simulink model "Simulator"  (R2024b)
settings: Solver=FixedStepAuto  StartTime=0.0  StopTime=Parameters.Simulink.sim_time_s  FixedStep=Parameters.Simulink.time_step_s  RelTol=1e-6
undefined symbols (not defined in the file): att_0, data, flight_mode, FLIGHT_MODE, id, joystick, Parameters, res, timestamp, traj_opt, wait_time_s
libraries: dspsigops x3, simulink x2, eeGeneralControl x2, px4uORBlib x2, vrlib x1, simulink_extras x1, aerolibanimutils x1, sharedtransform x1
(part 1 of 2)
settings Model: DataDictionary=simulink_data_types.sldd  Creator=thesa  LastModifiedBy=thesa
settings SolverCC: EnableFixedStepZeroCrossing=on
settings RTWCC: GPUComputeCapability=3.5

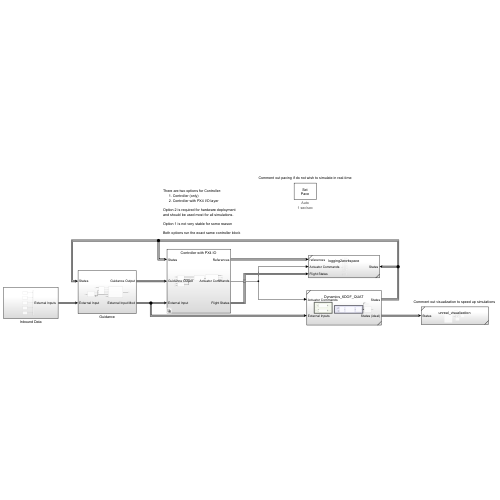
[thumbnail: Simulink's stored preview of the top-level diagram]
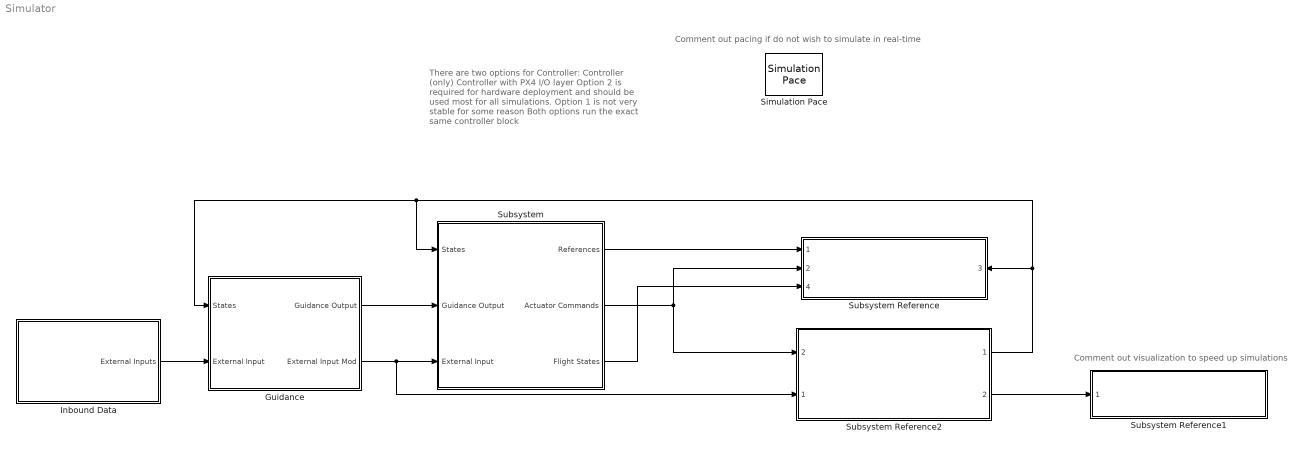
== system Simulator ==
  note: There are two options for Controller:
      | Controller (only)
      | Controller with PX4 I/O layer
      |
      | Option 2 is required for hardware deployment
      | and should be used most for all simulations.
      |
      | Option 1 is not very stable for some reason
      |
      | Both options run the exact same controller block
  note: Comment out pacing if do not wish to simulate in real-time
  note: Comment out visualization to speed up simulations
  Guidance : Subsystem
  Inbound Data : Subsystem
  Simulation Pace : aerolibanimutils/Simulation Pace  SimulationPace=1  SleepMode=Auto  OutputPaceError=off  SampleTime=-1
  Subsystem : Subsystem  Variant=on  VariantControlMode=label  VariantControl=Choice  LabelModeActiveChoice=Choice_1
  Subsystem Reference : Subsystem  ReferencedSubsystem=logging2workspace
      settings: PortSchema="{\"entries\":[{\"content\":{\"sides\":[{\"content\":{\"connectorIds\":[\"In1\",\"In2\",\"In4\"]},\"type\":\"ConnectorPlacement.EquallySpacedRectSide\",\"uuid\":\"47b0435c-4974-4dfb-aae6-6ca620e26367\"},{\"content\":{\"connectorIds\":[\"In3\"],\"side\":\"RIGHT\"},\"type\":\"ConnectorPlacement.EquallySpacedRectSide\",\"uuid\":\"e323305f-4ea2-4fd9-9ec2-838e165181fb\"},{\"content\":{\"side\":\"TOP\"},\"type\":\"ConnectorPlacement.EquallySpacedRectSide\",\"uuid\":\"bec00405-cbc9-4439-89df-ad1a7655b850\"}]},\"type\":\"ConnectorPlacement.EquallySpacedConnector\",\"uuid\":\"1e7e1f21-3d1e-40b5-a907-670aed2a63f6\"}],\"packageUris\":[\"http://schema.mathworks.com/mf0/Connector/R2020b\"],\"version\":\"1.0\"}"
  Subsystem Reference1 : Subsystem  ReferencedSubsystem=unreal_visualization
  Subsystem Reference2 : Subsystem  ReferencedSubsystem=Dynamics_6DOF_QUAT
      settings: PortSchema="{\"entries\":[{\"content\":{\"sides\":[{\"content\":{\"connectorIds\":[\"In2\",\"In1\"]},\"type\":\"ConnectorPlacement.EquallySpacedRectSide\",\"uuid\":\"67a10377-dfc9-4fe8-a62d-93af2914f52a\"},{\"content\":{\"connectorIds\":[\"Out1\",\"Out2\"],\"side\":\"RIGHT\"},\"type\":\"ConnectorPlacement.EquallySpacedRectSide\",\"uuid\":\"9c2068d6-d6c5-47ba-96fe-f41bc3930446\"},{\"content\":{\"side\":\"TOP\"},\"type\":\"ConnectorPlacement.EquallySpacedRectSide\",\"uuid\":\"c021d50f-d597-4e02-a45a-8416f053316a\"}]},\"type\":\"ConnectorPlacement.EquallySpacedConnector\",\"uuid\":\"5c77a6da-dceb-4faf-ad40-bce586c717c3\"}],\"packageUris\":[\"http://schema.mathworks.com/mf0/Connector/R2020b\"],\"version\":\"1.0\"}"
  wires:
  Inbound Data/1("External Inputs ") -> Guidance/2(External Input)
  Subsystem Reference2/1 -> Subsystem/1(States), Guidance/1(States), Subsystem Reference/3
  Subsystem/1(References) -> Subsystem Reference/1
  Subsystem/2(Actuator Commands) -> Subsystem Reference2/2, Subsystem Reference/2
  Subsystem/3(Flight States) -> Subsystem Reference/4
  Guidance/2(External Input Mod) -> Subsystem Reference2/1, Subsystem/3(External Input)
  Guidance/1(Guidance Output) -> Subsystem/2(Guidance Output)
  Subsystem Reference2/2 -> Subsystem Reference1/1

== system Simulator/Guidance ==
  States : Inport
  External Input : Inport  Port=2
  Guidance Initialization : Subsystem
  States1 : InportShadow
  Subsystem1 : Subsystem
  Subsystem2 : Subsystem  Variant=on  VariantControlMode=label  VariantControl=Choice  LabelModeActiveChoice=Choice
  Guidance Output : Outport
  External Input Mod : Outport  Port=2
  wires:
  Guidance Initialization/4(yaw_0) -> Subsystem2/4(yaw_0)
  Guidance Initialization/2(t) -> Subsystem2/2(time_since_start_of_traj)
  Subsystem2/1(trajectory) -> Guidance Output/1  "trajectory"
  Guidance Initialization/3("p_e_0 ") -> Subsystem2/3(p_e_0)
  States/1 -> Guidance Initialization/1(States)
  External Input/1 -> Subsystem1/1(External Input)
  Subsystem1/2(External Input Mod) -> Subsystem2/5(External Inputs), Guidance Initialization/2(External Input), External Input Mod/1
  Subsystem1/1(reset) -> Guidance Initialization/3(reset)
  States1/1 -> Subsystem2/6(States)
  Guidance Initialization/1(guidance_active) -> Subsystem2/1(guidance_active)

== system Simulator/Inbound Data ==
  Bus Creator3 : BusCreator  Inputs=5
  Subsystem1 : Subsystem
  Subsystem2 : Subsystem
  Subsystem3 : Subsystem
  Subsystem4 : Subsystem
  Subsystem5 : Subsystem
  "External Inputs " : Outport
  wires:
  Bus Creator3/1 -> "External Inputs "/1
  Subsystem1/1(Control Gains) -> Bus Creator3/2  "Control Gains"
  Subsystem2/1(Vehicle Parameters) -> Bus Creator3/1  "Vehicle Parameters"
  Subsystem3/1(Trajectory) -> Bus Creator3/4  "Trajectory"
  Subsystem4/1(Pilot Input) -> Bus Creator3/5  "Pilot Input"
  Subsystem5/1(Control Logic) -> Bus Creator3/3  "Control Logic"

== system Simulator/Subsystem ==
  States : Inport
  Guidance Output : Inport  Port=2
  External Input : Inport  Port=3
  Controller (only) : Subsystem  VariantControl=Controller (only)
  Controller with PX4 IO : Subsystem  VariantControl=Choice_1
  References : Outport
  Actuator Commands : Outport  Port=2
  Flight States : Outport  Port=3

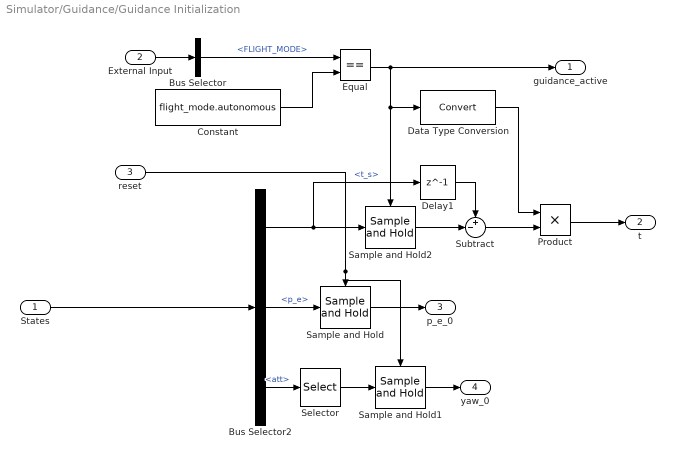
== system Simulator/Guidance/Guidance Initialization ==
  States : Inport
  External Input : Inport  Port=2
  reset : Inport  Port=3
  Bus Selector : BusSelector  OutputSignals=Pilot Input.FLIGHT_MODE
  Bus Selector2 : BusSelector  OutputSignals=t_s,p_e,att
  Constant : Constant  Value=flight_mode.autonomous
  Data Type Conversion : DataTypeConversion  SaturateOnIntegerOverflow=off  RndMeth=Floor
  Delay1 : Delay  DelayLength=1
  Equal : RelationalOperator  Operator===  OutDataTypeStr=boolean  RndMeth=Simplest  InputSameDT=off
  Product : Product
  Sample and Hold : dspsigops/Sample and Hold  trig=Rising edge  initCond=p_0  latchinput=off
  Sample and Hold1 : dspsigops/Sample and Hold  trig=Rising edge  initCond=att_0(3)  latchinput=off
  Sample and Hold2 : dspsigops/Sample and Hold  trig=Rising edge  initCond=0  latchinput=off
  Selector : Selector  InputPortWidth=3  IndexOptions=Index vector (dialog)  Indices=[3]  OutputSizes=1
  Subtract : Sum  Inputs=+-|
  guidance_active : Outport
  t : Outport  Port=2
  "p_e_0 " : Outport  Port=3
  yaw_0 : Outport  Port=4
  wires:
  Delay1/1 -> Subtract/1
  Subtract/1 -> Product/2
  Sample and Hold2/1 -> Subtract/2
  Bus Selector2/1 -> Delay1/1, Sample and Hold2/1  "<t_s>"
  Bus Selector2/3 -> Selector/1  "<att>"
  reset/1 -> Sample and Hold/Trigger, Sample and Hold1/Trigger
  States/1 -> Bus Selector2/1
  Bus Selector2/2 -> Sample and Hold/1  "<p_e>"
  Sample and Hold/1 -> "p_e_0 "/1
  Selector/1 -> Sample and Hold1/1
  Sample and Hold1/1 -> yaw_0/1
  External Input/1 -> Bus Selector/1
  Bus Selector/1 -> Equal/1  "<FLIGHT_MODE>"
  Constant/1 -> Equal/2
  Equal/1 -> guidance_active/1, Data Type Conversion/1, Sample and Hold2/Trigger
  Product/1 -> t/1
  Data Type Conversion/1 -> Product/1

== system Simulator/Guidance/Subsystem1 ==
  External Input : Inport
  Bus Assignment : BusAssignment  AssignedSignals=Pilot Input.FLIGHT_MODE
  Bus Selector : BusSelector  OutputSignals=Pilot Input.Parameters.time_step_s,Pilot Input.Parameters.AUTO_DELAY_S
  Bus Selector4 : BusSelector  OutputSignals=Pilot Input.FLIGHT_MODE
  Delay : Delay  DelayLength=1  InitialCondition=flight_mode.position_hold
  Delay1 : Delay  DelayLength=1
  Delay2 : Delay  DelayLength=1  InitialCondition=false
  Divide : Product  Inputs=*/
  MATLAB Function : MATLAB Function  TreatAsAtomicUnit=on
  reset : Outport
  External Input Mod : Outport  Port=2
  wires:
  MATLAB Function/1(current_mode) -> Delay/1
  External Input/1 -> Bus Assignment/1, Bus Selector4/1, Bus Selector/1
  Divide/1 -> MATLAB Function/4(wait_time)
  Bus Assignment/1 -> External Input Mod/1
  Bus Selector/2 -> Divide/1  "<AUTO_DELAY_S>"
  Bus Selector/1 -> Divide/2  "<time_step_s>"
  MATLAB Function/2(reset) -> Delay2/1
  MATLAB Function/3(timer) -> Delay1/1
  Delay/1 -> Bus Assignment/2, MATLAB Function/2("current_mode ")
  Bus Selector4/1 -> MATLAB Function/1(mode_request)  "<FLIGHT_MODE>"
  Delay1/1 -> MATLAB Function/3("timer ")
  Delay2/1 -> reset/1

== system Simulator/Guidance/Subsystem2 ==
  guidance_active : Inport
  time_since_start_of_traj : Inport  Port=2
  p_e_0 : Inport  Port=3
  yaw_0 : Inport  Port=4
  External Inputs : Inport  Port=5
  States : Inport  Port=6
  Step input : Subsystem  VariantControl=Choice_1
  minimum_snap : Subsystem  VariantControl=Choice
  trajectory : Outport

== system Simulator/Inbound Data/Subsystem1 ==
  " K-matrix control (LQR, H-inf, etc.)" : Subsystem
  Bus Creator2 : BusCreator  Inputs=9
  Constant1 : Constant  Value=Parameters.Control.Gains.K_omega_dot
  Constant13 : Constant  Value=Parameters.Control.Gains.K_omega
  Constant18 : Constant  Value=Parameters.Control.Gains.K_pos_int
  Constant2 : Constant  Value=Parameters.Control.Gains.K_omega_I
  Constant6 : Constant  Value=Parameters.Control.Gains.K_pos
  Constant7 : Constant  Value=Parameters.Control.Gains.K_vel
  Constant8 : Constant  Value=Parameters.Control.Gains.K_att
  Constant9 : Constant  Value=Parameters.Control.Gains.K_acc
  Control Gains : Outport
  wires:
  Constant7/1 -> Bus Creator2/3  "K_vel"
  Constant6/1 -> Bus Creator2/1  "K_pos"
  Constant13/1 -> Bus Creator2/6  "K_omega"
  Bus Creator2/1 -> Control Gains/1  "Control Gains"
  Constant18/1 -> Bus Creator2/2  "K_pos_int"
  Constant9/1 -> Bus Creator2/4  "K_acc"
  Constant8/1 -> Bus Creator2/5  "K_att"
  " K-matrix control (LQR, H-inf, etc.)"/1(K_matrix_control) -> Bus Creator2/9  "K_matrix_control"
  Constant1/1 -> Bus Creator2/8  "K_omega_dot"
  Constant2/1 -> Bus Creator2/7  "K_omega_I"

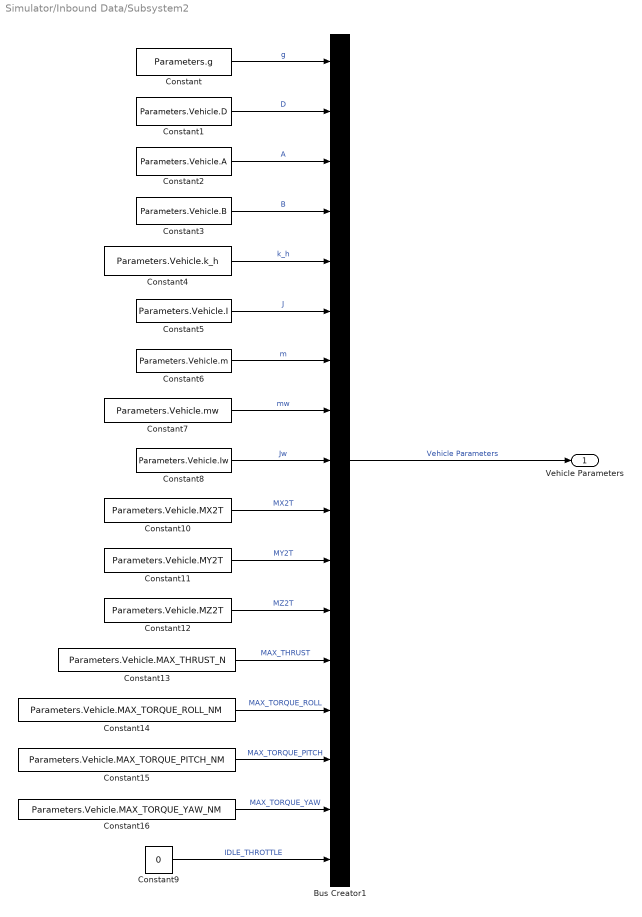
== system Simulator/Inbound Data/Subsystem2 ==
  Bus Creator1 : BusCreator  Inputs=17
  Constant : Constant  Value=Parameters.g
  Constant1 : Constant  Value=Parameters.Vehicle.D
  Constant10 : Constant  Value=Parameters.Vehicle.MX2T
  Constant11 : Constant  Value=Parameters.Vehicle.MY2T
  Constant12 : Constant  Value=Parameters.Vehicle.MZ2T
  Constant13 : Constant  Value=Parameters.Vehicle.MAX_THRUST_N
  Constant14 : Constant  Value=Parameters.Vehicle.MAX_TORQUE_ROLL_NM
  Constant15 : Constant  Value=Parameters.Vehicle.MAX_TORQUE_PITCH_NM
  Constant16 : Constant  Value=Parameters.Vehicle.MAX_TORQUE_YAW_NM
  Constant2 : Constant  Value=Parameters.Vehicle.A
  Constant3 : Constant  Value=Parameters.Vehicle.B
  Constant4 : Constant  Value=Parameters.Vehicle.k_h
  Constant5 : Constant  Value=Parameters.Vehicle.I
  Constant6 : Constant  Value=Parameters.Vehicle.m
  Constant7 : Constant  Value=Parameters.Vehicle.mw
  Constant8 : Constant  Value=Parameters.Vehicle.Iw
  Constant9 : Constant  Value=0
  Vehicle Parameters : Outport
  wires:
  Constant5/1 -> Bus Creator1/6  "J"
  Constant3/1 -> Bus Creator1/4  "B"
  Constant/1 -> Bus Creator1/1  "g"
  Constant1/1 -> Bus Creator1/2  "D"
  Constant2/1 -> Bus Creator1/3  "A"
  Constant4/1 -> Bus Creator1/5  "k_h"
  Bus Creator1/1 -> Vehicle Parameters/1  "Vehicle Parameters"
  Constant6/1 -> Bus Creator1/7  "m"
  Constant7/1 -> Bus Creator1/8  "mw"
  Constant8/1 -> Bus Creator1/9  "Jw"
  Constant10/1 -> Bus Creator1/10  "MX2T"
  Constant11/1 -> Bus Creator1/11  "MY2T"
  Constant12/1 -> Bus Creator1/12  "MZ2T"
  Constant13/1 -> Bus Creator1/13  "MAX_THRUST"
  Constant14/1 -> Bus Creator1/14  "MAX_TORQUE_ROLL"
  Constant15/1 -> Bus Creator1/15  "MAX_TORQUE_PITCH"
  Constant16/1 -> Bus Creator1/16  "MAX_TORQUE_YAW"
  Constant9/1 -> Bus Creator1/17  "IDLE_THROTTLE"

== system Simulator/Inbound Data/Subsystem3 ==
  Trajectory Solution : Subsystem  Variant=on  VariantControlMode=label  VariantControl=Choice  LabelModeActiveChoice=Choice
  Trajectory : Outport
  wires:
  Trajectory Solution/1(Trajectory) -> Trajectory/1

== system Simulator/Inbound Data/Subsystem4 ==
  Bus Creator4 : BusCreator  Inputs=4
  Subsystem : Subsystem
  Subsystem1 : Subsystem
  Pilot Input : Outport
  wires:
  Subsystem/1(sticks) -> Bus Creator4/1  "Sticks"
  Bus Creator4/1 -> Pilot Input/1  "Pilot Input"
  Subsystem1/1(Parameters) -> Bus Creator4/4  "Parameters"
  Subsystem/2(FLIGHT_MODE) -> Bus Creator4/2  "FLIGHT_MODE"
  Subsystem/3(ARMED) -> Bus Creator4/3  "ARMED"

== system Simulator/Inbound Data/Subsystem5 ==
  Bus Creator2 : BusCreator  Inputs=5
  Constant18 : Constant  Value=Parameters.Control.Logic.MAX_VEL_VERTICAL
  Constant6 : Constant  Value=Parameters.Control.Logic.MAX_VEL_HORIZONTAL
  Constant7 : Constant  Value=Parameters.Control.Logic.MAX_TILT
  Constant8 : Constant  Value=Parameters.Control.Logic.MAX_TH
  Constant9 : Constant  Value=Parameters.Control.Logic.MIN_TH
  Degrees to Radians : simulink_extras/Transformations/Degrees to Radians
  Control Logic : Outport
  wires:
  Constant8/1 -> Bus Creator2/5  "MAX_TH"
  Constant9/1 -> Bus Creator2/4  "MIN_TH"
  Constant18/1 -> Bus Creator2/2  "MAX_VEL_VERTICAL"
  Bus Creator2/1 -> Control Logic/1  "Control Logic"
  Constant6/1 -> Bus Creator2/1  "MAX_VEL_HORIZONTAL"
  Constant7/1 -> Degrees to Radians/1
  Degrees to Radians/1 -> Bus Creator2/3  "MAX_TILT_RAD"

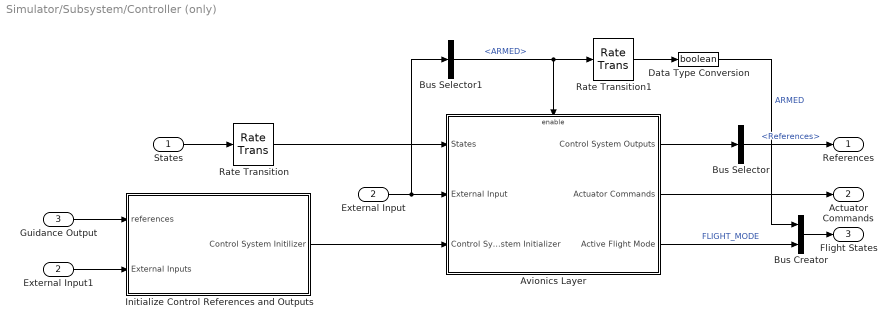
== system Simulator/Subsystem/Controller (only) ==
  States : Inport
  External Input : Inport  Port=2
  Guidance Output : Inport  Port=3
  Avionics Layer : Subsystem  TreatAsAtomicUnit=on
  Bus Creator : BusCreator  Inputs=2
  Bus Selector : BusSelector  OutputSignals=Control System Outputs.References
  Bus Selector1 : BusSelector  OutputSignals=Pilot Input.ARMED
  Data Type Conversion : DataTypeConversion  OutDataTypeStr=boolean  SaturateOnIntegerOverflow=off  RndMeth=Floor
  External Input1 : InportShadow  Port=2
  Initialize Control References and Outputs : Subsystem
  Rate Transition : RateTransition  OutPortSampleTime=Parameters.Simulink.time_step_s
  Rate Transition1 : RateTransition  OutPortSampleTime=Parameters.Simulink.time_step_s
  References : Outport
  Actuator Commands : Outport  Port=2
  Flight States : Outport  Port=3
  wires:
  Avionics Layer/1(Control System Outputs) -> Bus Selector/1
  Avionics Layer/2(Actuator Commands) -> Actuator Commands/1
  States/1 -> Rate Transition/1
  Bus Creator/1 -> Flight States/1
  Avionics Layer/3(Active Flight Mode) -> Bus Creator/2  "FLIGHT_MODE"
  Data Type Conversion/1 -> Bus Creator/1  "ARMED"
  Initialize Control References and Outputs/1(Control System Initilizer) -> Avionics Layer/3(Control System Initializer)
  Guidance Output/1 -> Initialize Control References and Outputs/1(references)
  External Input1/1 -> Initialize Control References and Outputs/2(External Inputs)
  Bus Selector/1 -> References/1  "<References>"
  External Input/1 -> Bus Selector1/1, Avionics Layer/2(External Input)
  Bus Selector1/1 -> Avionics Layer/Enable, Rate Transition1/1  "<ARMED>"
  Rate Transition/1 -> Avionics Layer/1(States)
  Rate Transition1/1 -> Data Type Conversion/1

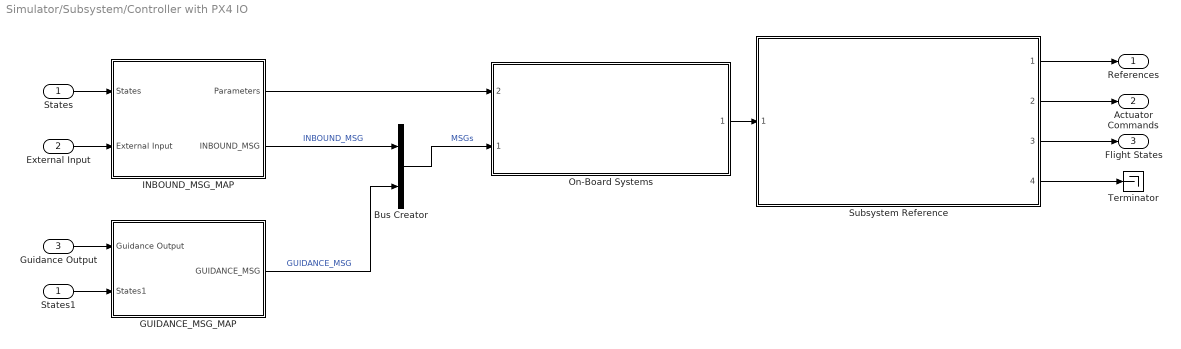
== system Simulator/Subsystem/Controller with PX4 IO ==
  States : Inport
  External Input : Inport  Port=2
  Guidance Output : Inport  Port=3
  Bus Creator : BusCreator  Inputs=2
  GUIDANCE_MSG_MAP : Subsystem
  INBOUND_MSG_MAP : Subsystem
  On-Board Systems : Subsystem  ReferencedSubsystem=PX4IO_Layer
      settings: PortSchema="{\"entries\":[{\"content\":{\"sides\":[{\"content\":{\"connectorIds\":[\"In2\",\"In1\"]},\"type\":\"ConnectorPlacement.EquallySpacedRectSide\",\"uuid\":\"a5730cf6-2872-4e25-8304-8f22dd734b05\"},{\"content\":{\"connectorIds\":[\"Out1\"],\"side\":\"RIGHT\"},\"type\":\"ConnectorPlacement.EquallySpacedRectSide\",\"uuid\":\"3d39f402-1208-4784-94d4-56674b3fcefd\"},{\"content\":{\"side\":\"TOP\"},\"type\":\"ConnectorPlacement.EquallySpacedRectSide\",\"uuid\":\"c866c1ba-d1e0-4217-90d9-3f868bb9a07c\"}]},\"type\":\"ConnectorPlacement.EquallySpacedConnector\",\"uuid\":\"0dae0d84-579d-4ec0-afcf-2d35a51e434b\"}],\"packageUris\":[\"http://schema.mathworks.com/mf0/Connector/R2020b\"],\"version\":\"1.0\"}"
  States1 : InportShadow
  Subsystem Reference : Subsystem  ReferencedSubsystem=OUTBOUND_MSG_UNMAP
  Terminator : Terminator
  References : Outport
  Actuator Commands : Outport  Port=2
  Flight States : Outport  Port=3
  wires:
  INBOUND_MSG_MAP/1(Parameters) -> On-Board Systems/2
  States/1 -> INBOUND_MSG_MAP/1(States)
  On-Board Systems/1 -> Subsystem Reference/1
  INBOUND_MSG_MAP/2(INBOUND_MSG) -> Bus Creator/1  "INBOUND_MSG"
  Subsystem Reference/2 -> Actuator Commands/1
  Subsystem Reference/1 -> References/1
  External Input/1 -> INBOUND_MSG_MAP/2(External Input)
  Subsystem Reference/3 -> Flight States/1
  Bus Creator/1 -> On-Board Systems/1  "MSGs"
  Guidance Output/1 -> GUIDANCE_MSG_MAP/1(Guidance Output)
  States1/1 -> GUIDANCE_MSG_MAP/2(States1)
  GUIDANCE_MSG_MAP/1(GUIDANCE_MSG) -> Bus Creator/2  "GUIDANCE_MSG"
  Subsystem Reference/4 -> Terminator/1

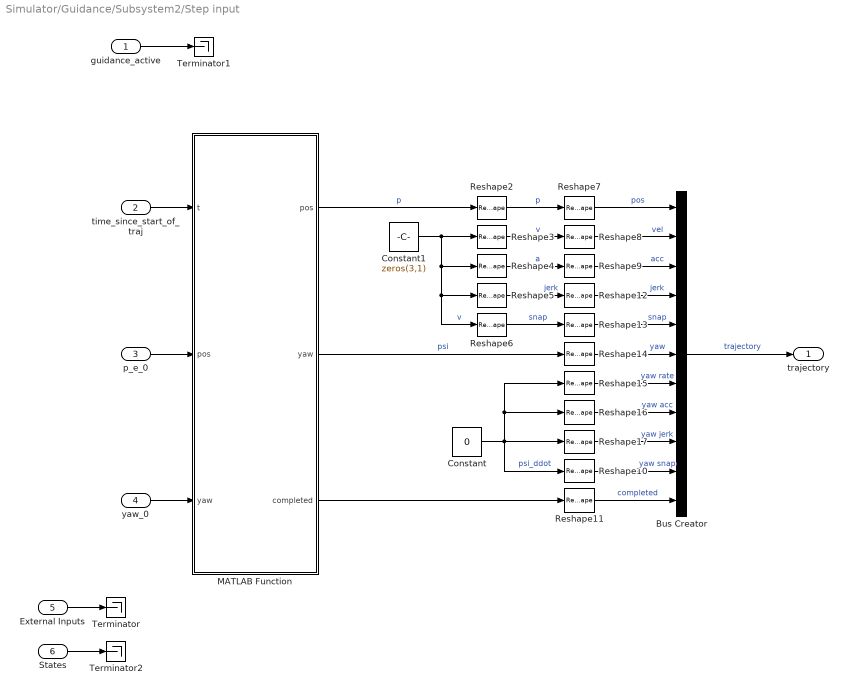
== system Simulator/Guidance/Subsystem2/Step input ==
  guidance_active : Inport
  time_since_start_of_traj : Inport  Port=2
  p_e_0 : Inport  Port=3
  yaw_0 : Inport  Port=4
  External Inputs : Inport  Port=5
  States : Inport  Port=6
  Bus Creator : BusCreator  Inputs=11
  Constant : Constant  Value=0
  Constant1 : Constant  Value=zeros(3,1)
  MATLAB Function : MATLAB Function  TreatAsAtomicUnit=on
  Reshape{7..17} (11 alike) : Reshape
  Reshape{2..6} (5 alike) : Reshape  OutputDimensionality=Column vector (2-D)
  Terminator : Terminator
  Terminator1 : Terminator
  Terminator2 : Terminator
  trajectory : Outport
  wires:
  Reshape4/1 -> Reshape9/1  "a"
  Reshape12/1 -> Bus Creator/4  "jerk"
  Constant1/1 -> Reshape6/1, Reshape5/1, Reshape4/1, Reshape3/1  "v"
  Reshape6/1 -> Reshape13/1  "snap"
  Reshape13/1 -> Bus Creator/5  "snap"
  Reshape7/1 -> Bus Creator/1  "pos"
  Reshape16/1 -> Bus Creator/8  "yaw acc"
  MATLAB Function/1(pos) -> Reshape2/1  "p"
  MATLAB Function/3(completed) -> Reshape11/1
  Reshape15/1 -> Bus Creator/7  "yaw rate"
  Reshape5/1 -> Reshape12/1  "jerk"
  Constant/1 -> Reshape10/1, Reshape15/1, Reshape16/1, Reshape17/1  "psi_ddot"
  Reshape14/1 -> Bus Creator/6  "yaw"
  MATLAB Function/2(yaw) -> Reshape14/1  "psi"
  Reshape10/1 -> Bus Creator/10  "yaw snap"
  Reshape2/1 -> Reshape7/1  "p"
  Reshape9/1 -> Bus Creator/3  "acc"
  Reshape3/1 -> Reshape8/1  "v"
  Bus Creator/1 -> trajectory/1  "trajectory"
  Reshape17/1 -> Bus Creator/9  "yaw jerk"
  Reshape8/1 -> Bus Creator/2  "vel"
  Reshape11/1 -> Bus Creator/11  "completed"
  External Inputs/1 -> Terminator/1
  yaw_0/1 -> MATLAB Function/3("yaw ")
  p_e_0/1 -> MATLAB Function/2("pos ")
  time_since_start_of_traj/1 -> MATLAB Function/1(t)
  guidance_active/1 -> Terminator1/1
  States/1 -> Terminator2/1

== system Simulator/Guidance/Subsystem2/minimum_snap ==
  guidance_active : Inport
  time_since_start_of_traj : Inport  Port=2
  p_e_0 : Inport  Port=3
  yaw_0 : Inport  Port=4
  External Inputs : Inport  Port=5
  States : Inport  Port=6
  Bus Selector1 : BusSelector  OutputSignals=Trajectory
  Mux : Mux  Inputs=2
  Reshape : Reshape
  Reshape1 : Reshape
  Subsystem : Subsystem  Variant=on  VariantControlMode=label  VariantControl=Choice  LabelModeActiveChoice=Choice
  trajectory : Outport
  wires:
  Subsystem/1(trajectory) -> trajectory/1  "trajectory"
  External Inputs/1 -> Bus Selector1/1
  time_since_start_of_traj/1 -> Subsystem/2(time_since_start_of_traj)
  Mux/1 -> Subsystem/5(waypoints_offset_0)  "waypoints_offset_0"
  Reshape1/1 -> Mux/2
  yaw_0/1 -> Reshape1/1
  p_e_0/1 -> Reshape/1
  Reshape/1 -> Mux/1
  Bus Selector1/1 -> Subsystem/3(Trajectory)  "<Trajectory>"
  States/1 -> Subsystem/4(States)
  guidance_active/1 -> Subsystem/1(guidance_active)

== system Simulator/Inbound Data/Subsystem1/ K-matrix control (LQR, H-inf, etc.) ==
  Bus Creator : BusCreator  Inputs=3
  Constant1 : Constant  Value=Parameters.K_Control.K
  Constant2 : Constant  Value=Parameters.K_Control.EN
  Constant3 : Constant  Value=Parameters.K_Control.K_pos_int
  K_matrix_control : Outport
  wires:
  Bus Creator/1 -> K_matrix_control/1  "K_matrix_control"
  Constant1/1 -> Bus Creator/2  "K"
  Constant2/1 -> Bus Creator/1  "EN"
  Constant3/1 -> Bus Creator/3  "K_pos_int"

== system Simulator/Inbound Data/Subsystem3/Trajectory Solution ==
  Call solver : Subsystem  VariantControl=Choice_1
  Static : Subsystem  VariantControl=Choice
  Trajectory : Outport

== system Simulator/Inbound Data/Subsystem4/Subsystem ==
  Bus Creator4 : BusCreator  Inputs=4
  Display{1..5} (5 alike) : Display
  Subsystem1 : Subsystem  Variant=on  VariantControlMode=label  VariantControl=Choice  LabelModeActiveChoice=Choice_1
  sticks : Outport
  FLIGHT_MODE : Outport  Port=2
  ARMED : Outport  Port=3
  wires:
  Bus Creator4/1 -> sticks/1
  Subsystem1/1(roll_stick) -> Bus Creator4/1, Display2/1
  Subsystem1/2(pitch_stick) -> Bus Creator4/2, Display3/1
  Subsystem1/3(yaw_stick) -> Display4/1, Bus Creator4/3
  Subsystem1/4(Throttle_stick) -> Display5/1, Bus Creator4/4
  Subsystem1/5(FLIGHT_MODE) -> FLIGHT_MODE/1, Display1/1
  Subsystem1/6(ARMED) -> ARMED/1

== system Simulator/Inbound Data/Subsystem4/Subsystem1 ==
  Bus Creator : BusCreator  Inputs=9
  Constant : Constant  Value=Parameters.Control.Gains.MANUAL_ROLL_STICK_GAIN
  Constant1 : Constant  Value=Parameters.Control.Gains.MANUAL_PITCH_STICK_GAIN
  Constant2 : Constant  Value=Parameters.Control.Gains.MANUAL_YAW_RATE_STICK_GAIN
  Constant3 : Constant  Value=Parameters.Control.Gains.MANUAL_THRUST_STICK_GAIN
  Constant4 : Constant  Value=Parameters.Control.Gains.VELOCITY_XY_STICK_GAIN
  Constant5 : Constant  Value=Parameters.Control.Gains.VELOCITY_Z_STICK_GAIN
  Constant6 : Constant  Value=Parameters.Control.Logic.AUTO_DELAY_S
  Constant7 : Constant  Value=Parameters.Simulink.time_step_s
  Constant8 : Constant  Value=Parameters.Control.Logic.GEN_FF_T_TAU
  Parameters : Outport
  wires:
  Constant/1 -> Bus Creator/1  "MANUAL_ROLL_STICK_GAIN"
  Bus Creator/1 -> Parameters/1  "Parameters"
  Constant1/1 -> Bus Creator/2  "MANUAL_PITCH_STICK_GAIN"
  Constant2/1 -> Bus Creator/3  "MANUAL_YAW_RATE_STICK_GAIN"
  Constant3/1 -> Bus Creator/4  "MANUAL_THRUST_STICK_GAIN"
  Constant4/1 -> Bus Creator/5  "VELOCITY_XY_STICK_GAIN"
  Constant5/1 -> Bus Creator/6  "VELOCITY_Z_STICK_GAIN"
  Constant6/1 -> Bus Creator/7  "AUTO_DELAY_S"
  Constant7/1 -> Bus Creator/8  "time_step_s"
  Constant8/1 -> Bus Creator/9  "GEN_FF_T_TAU"

== system Simulator/Subsystem/Controller (only)/Avionics Layer ==
  States : Inport
  External Input : Inport  Port=2
  Control System Initializer : Inport  Port=3
  Enable : EnablePort  StatesWhenEnabling=reset  PropagateVarSize=During execution
  Subsystem Reference : Subsystem  ReferencedSubsystem=Controller
  Control System Outputs : Outport
  Actuator Commands : Outport  Port=2
  Active Flight Mode : Outport  Port=3
  wires:
  Subsystem Reference/1 -> Control System Outputs/1
  Subsystem Reference/2 -> Actuator Commands/1
  States/1 -> Subsystem Reference/1
  External Input/1 -> Subsystem Reference/2
  Subsystem Reference/3 -> Active Flight Mode/1
  Control System Initializer/1 -> Subsystem Reference/3

== system Simulator/Subsystem/Controller (only)/Initialize Control References and Outputs ==
  references : Inport
  External Inputs : Inport  Port=2
  Bus Creator : BusCreator  Inputs=2
  Bus Creator2 : BusCreator  Inputs=2
  Bus Selector1 : BusSelector  OutputSignals=pos,vel,acc,jerk,snap,yaw,yaw rate,yaw acc,completed
  Bus Selector3 : BusSelector  OutputSignals=Vehicle Parameters.g,Vehicle Parameters.m
  Constant : Constant  Value=zeros(3,1)
  Constant1 : Constant  Value=zeros(1,2)
  Divide : Product  Inputs=**
  Reshape : Reshape  OutputDimensionality=Column vector (2-D)
  Reshape1 : Reshape
  Subsystem1 : Subsystem
  Control System Initilizer : Outport
  wires:
  Bus Selector1/9 -> Subsystem1/12(completed)  "<completed>"
  Reshape1/1 -> Subsystem1/9(roll_pitch_ref), Subsystem1/10(pq_ref)
  Bus Selector1/8 -> Subsystem1/8(yaw_acc_ref)  "<yaw acc>"
  Bus Selector1/7 -> Subsystem1/7(yaw_rate_ref)  "<yaw rate>"
  Bus Selector1/6 -> Subsystem1/6(yaw_ref)  "<yaw>"
  Bus Selector1/5 -> Subsystem1/5(s_e_ref)  "<snap>"
  Bus Selector1/4 -> Subsystem1/4(j_e_ref)  "<jerk>"
  Bus Selector1/3 -> Subsystem1/3(a_e_ref)  "<acc>"
  Bus Selector1/2 -> Subsystem1/2(v_e_ref)  "<vel>"
  Bus Selector1/1 -> Subsystem1/1(p_e_ref)  "<pos>"
  Bus Selector3/2 -> Divide/2  "<m>"
  Reshape/1 -> Bus Creator2/2  "Tau"
  Bus Creator2/1 -> Bus Creator/2  "Control Outputs"
  Constant/1 -> Reshape/1
  Divide/1 -> Subsystem1/11(T), Bus Creator2/1  "T"
  Bus Creator/1 -> Control System Initilizer/1
  External Inputs/1 -> Bus Selector3/1
  Bus Selector3/1 -> Divide/1  "<g>"
  references/1 -> Bus Selector1/1
  Subsystem1/1(references) -> Bus Creator/1  "References"
  Constant1/1 -> Reshape1/1

== system Simulator/Subsystem/Controller with PX4 IO/GUIDANCE_MSG_MAP ==
  Guidance Output : Inport
  States1 : Inport  Port=2
  Bus Assignment : BusAssignment  AssignedSignals=timestamp,id,data
  Bus Selector : BusSelector  OutputSignals=t_s
  Bus Selector1 : BusSelector  OutputSignals=pos,vel,acc,jerk,snap,yaw,yaw rate,yaw acc,yaw jerk,yaw snap,completed
  Constant2 : Constant  Value=uint16(150)  OutDataTypeStr=uint16
  Data Type Conversion : DataTypeConversion  SaturateOnIntegerOverflow=off  RndMeth=Floor
  Data Type Conversion2 : DataTypeConversion  OutDataTypeStr=single  RndMeth=Round  SaturateOnIntegerOverflow=off
  Gain : Gain  Gain=1E6
  MATLAB Function : MATLAB Function  TreatAsAtomicUnit=on
  PX4 uORB Message : px4uORBlib/PX4 uORB Message  uORBTopic=DebugArray  SampleTime=inf  selectInstance=debug_array
  Reshape : Reshape
  GUIDANCE_MSG : Outport
  wires:
  Reshape/1 -> Bus Assignment/4
  Gain/1 -> Data Type Conversion/1
  Constant2/1 -> Bus Assignment/3
  Data Type Conversion/1 -> Bus Assignment/2
  States1/1 -> Bus Selector/1
  PX4 uORB Message/1 -> Bus Assignment/1
  Bus Selector/1 -> Gain/1  "<t_s>"
  Bus Assignment/1 -> GUIDANCE_MSG/1  "GUIDANCE_MSG"
  MATLAB Function/1(GUIDANCE_DATA_MSG) -> Data Type Conversion2/1
  Data Type Conversion2/1 -> Reshape/1
  Guidance Output/1 -> Bus Selector1/1
  Bus Selector1/1 -> MATLAB Function/1(pos)  "<pos>"
  Bus Selector1/2 -> MATLAB Function/2(vel)  "<vel>"
  Bus Selector1/3 -> MATLAB Function/3(acc)  "<acc>"
  Bus Selector1/4 -> MATLAB Function/4(jerk)  "<jerk>"
  Bus Selector1/5 -> MATLAB Function/5(snap)  "<snap>"
  Bus Selector1/6 -> MATLAB Function/6(yaw)  "<yaw>"
  Bus Selector1/7 -> MATLAB Function/7(yaw_rate)  "<yaw rate>"
  Bus Selector1/8 -> MATLAB Function/8(yaw_acc)  "<yaw acc>"
  Bus Selector1/11 -> MATLAB Function/11(completed)  "<completed>"
  Bus Selector1/10 -> MATLAB Function/10(yaw_snap)  "<yaw snap>"
  Bus Selector1/9 -> MATLAB Function/9(yaw_jerk)  "<yaw jerk>"

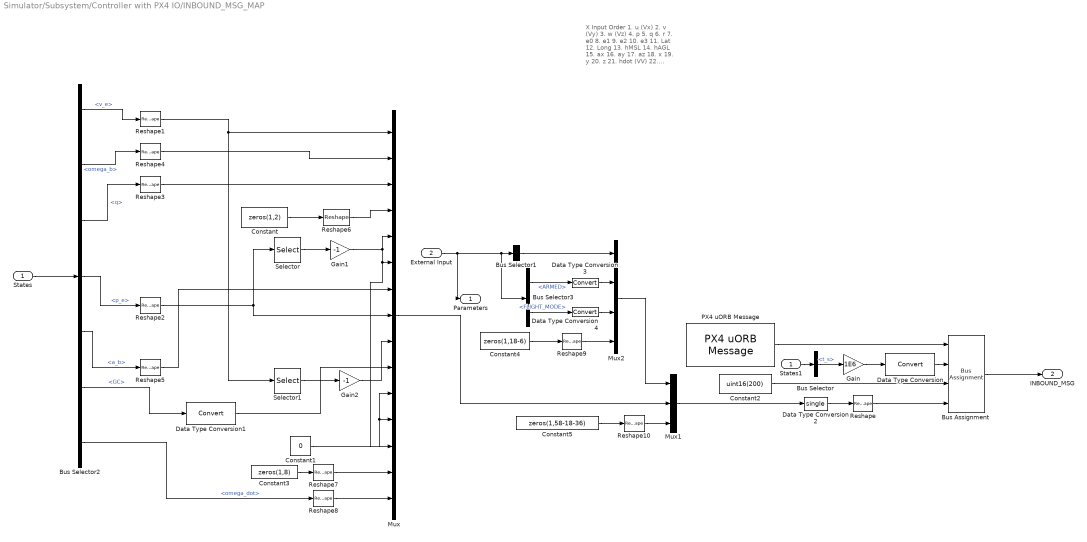
== system Simulator/Subsystem/Controller with PX4 IO/INBOUND_MSG_MAP ==
  note: X Input Order
      | 1. u (Vx)
      | 2. v (Vy)
      | 3. w (Vz)
      | 4. p
      | 5. q
      | 6. r
      | 7. e0
      | 8. e1
      | 9. e2
      | 10. e3
      | 11. Lat
      | 12. Long
      | 13. hMSL
      | 14. hAGL
      | 15. ax
      | 16. ay
      | 17. az
      | 18. x
      | 19. y
      | 20. z
      | 21. hdot (VV)
      | 22. GCFlag
      | 23. TAS
      | 24. EAS
      | 25. LiDAR
  States : Inport
  External Input : Inport  Port=2
  Bus Assignment : BusAssignment  AssignedSignals=timestamp,id,data
  Bus Selector : BusSelector  OutputSignals=t_s
  Bus Selector1 : BusSelector  OutputSignals=Pilot Input.Sticks.roll_stick,Pilot Input.Sticks.pitch_stick,Pilot Input.Sticks.yaw_stick,Pilot Input.Sticks.Throttle_stick  OutputAsBus=on
  Bus Selector2 : BusSelector  OutputSignals=v_e,omega_b,q,p_e,a_b,GC,omega_dot
  Bus Selector3 : BusSelector  OutputSignals=Pilot Input.ARMED,Pilot Input.FLIGHT_MODE
  Constant : Constant  Value=zeros(1,2)
  Constant1 : Constant  Value=0
  Constant2 : Constant  Value=uint16(200)  OutDataTypeStr=uint16
  Constant3 : Constant  Value=zeros(1,8)
  Constant4 : Constant  Value=zeros(1,18-6)
  Constant5 : Constant  Value=zeros(1,58-18-36)
  Data Type Conversion{,1,3..4} (4 alike) : DataTypeConversion  SaturateOnIntegerOverflow=off  RndMeth=Floor
  Data Type Conversion2 : DataTypeConversion  OutDataTypeStr=single  RndMeth=Round  SaturateOnIntegerOverflow=off
  Gain : Gain  Gain=1E6
  Gain1 : Gain  Gain=-1
  Gain2 : Gain  Gain=-1
  Mux : Mux  Inputs=15
  Mux1 : Mux  Inputs=3
  Mux2 : Mux
  PX4 uORB Message : px4uORBlib/PX4 uORB Message  uORBTopic=DebugArray  SampleTime=inf  selectInstance=debug_array
  Reshape : Reshape  OutputDimensionality=Row vector (2-D)
  Reshape{1..10} (10 alike) : Reshape
  Selector : Selector  InputPortWidth=3  IndexOptions=Index vector (dialog)  Indices=[3]  OutputSizes=1
  Selector1 : Selector  InputPortWidth=3  IndexOptions=Index vector (dialog)  Indices=[3]  OutputSizes=1
  States1 : InportShadow
  Parameters : Outport
  INBOUND_MSG : Outport  Port=2
  wires:
  Bus Assignment/1 -> INBOUND_MSG/1
  External Input/1 -> Parameters/1, Bus Selector3/1, Bus Selector1/1
  PX4 uORB Message/1 -> Bus Assignment/1
  Constant2/1 -> Bus Assignment/3
  Data Type Conversion/1 -> Bus Assignment/2
  Data Type Conversion2/1 -> Reshape/1
  Reshape/1 -> Bus Assignment/4
  States/1 -> Bus Selector2/1
  Bus Selector2/1 -> Reshape1/1  "<v_e>"
  Bus Selector2/4 -> Reshape2/1  "<p_e>"
  Bus Selector2/3 -> Reshape3/1  "<q>"
  Bus Selector2/2 -> Reshape4/1  "<omega_b>"
  Bus Selector2/5 -> Reshape5/1  "<a_b>"
  Reshape1/1 -> Selector1/1, Mux/1
  Reshape3/1 -> Mux/3
  Constant/1 -> Reshape6/1
  Reshape6/1 -> Mux/4
  Selector/1 -> Gain1/1
  Gain1/1 -> Mux/13, Mux/6, Mux/5
  Reshape2/1 -> Mux/8, Selector/1
  Reshape5/1 -> Mux/7
  Selector1/1 -> Gain2/1
  Gain2/1 -> Mux/9
  Constant1/1 -> Mux/12, Mux/11
  Reshape4/1 -> Mux/2
  Mux/1 -> Mux1/2
  States1/1 -> Bus Selector/1
  Bus Selector/1 -> Gain/1  "<t_s>"
  Gain/1 -> Data Type Conversion/1
  Bus Selector2/6 -> Data Type Conversion1/1  "<GC>"
  Data Type Conversion1/1 -> Mux/10
  Mux1/1 -> Data Type Conversion2/1
  Bus Selector1/1 -> Mux2/1
  Constant3/1 -> Reshape7/1
  Reshape7/1 -> Mux/14
  Bus Selector2/7 -> Reshape8/1  "<omega_dot>"
  Reshape8/1 -> Mux/15
  Constant4/1 -> Reshape9/1
  Mux2/1 -> Mux1/1
  Reshape9/1 -> Mux2/4
  Constant5/1 -> Reshape10/1
  Reshape10/1 -> Mux1/3
  Bus Selector3/1 -> Data Type Conversion3/1  "<ARMED>"
  Bus Selector3/2 -> Data Type Conversion4/1  "<FLIGHT_MODE>"
  Data Type Conversion3/1 -> Mux2/2
  Data Type Conversion4/1 -> Mux2/3

== system Simulator/Guidance/Subsystem2/minimum_snap/Subsystem ==
  guidance_active : Inport
  time_since_start_of_traj : Inport  Port=2
  Trajectory : Inport  Port=3
  States : Inport  Port=4
  waypoints_offset_0 : Inport  Port=5
  re-solve trajectory : Subsystem  VariantControl=Choice_1
  use static solution : Subsystem  VariantControl=Choice
  trajectory : Outport

== system Simulator/Inbound Data/Subsystem3/Trajectory Solution/Call solver ==
  Constant : Constant  Value=false
  Constant1 : Constant  Value=traj_opt
  Delay : Delay  DelayLength=1  InitialCondition=true
  Enabled Subsystem : Subsystem  TreatAsAtomicUnit=on
  Trajectory : Outport
  wires:
  Constant/1 -> Delay/1
  Constant1/1 -> Enabled Subsystem/1(trajectory_id)
  Delay/1 -> Enabled Subsystem/Enable
  Enabled Subsystem/1(Trajectory) -> Trajectory/1

== system Simulator/Inbound Data/Subsystem3/Trajectory Solution/Static ==
  note: res.n_dim = this.n_dim;
      | res.n_dim_src = this.n_dim_src;
      | res.n_dim_ids = this.n_dim_ids;
      | res.N_segments = this.N_segments;
  Bus Creator : BusCreator  Inputs=6
  Constant11 : Constant  Value=res.minsnap_set.T
  Constant12 : Constant  Value=res.minsnap_set.pp
  Constant14 : Constant  Value=res.minsnap_set.n_dim
  Constant15 : Constant  Value=res.minsnap_set.n_dim_src
  Constant16 : Constant  Value=res.minsnap_set.n_dim_ids
  Constant17 : Constant  Value=res.minsnap_set.N_segments
  Trajectory : Outport
  wires:
  Constant17/1 -> Bus Creator/6  "N_Segments"
  Constant14/1 -> Bus Creator/3  "n_dim"
  Constant16/1 -> Bus Creator/5  "n_dim_ids"
  Constant11/1 -> Bus Creator/1  "T"
  Constant12/1 -> Bus Creator/2  "coefs"
  Bus Creator/1 -> Trajectory/1  "Trajectory"
  Constant15/1 -> Bus Creator/4  "n_dim_src"

== system Simulator/Inbound Data/Subsystem4/Subsystem/Subsystem1 ==
  Disabled : Subsystem  VariantControl=Choice_1
  Joytick : Subsystem  VariantControl=Choice
  Sliders : Subsystem  VariantControl=Choice_2
  roll_stick : Outport
  pitch_stick : Outport  Port=2
  yaw_stick : Outport  Port=3
  Throttle_stick : Outport  Port=4
  FLIGHT_MODE : Outport  Port=5
  ARMED : Outport  Port=6

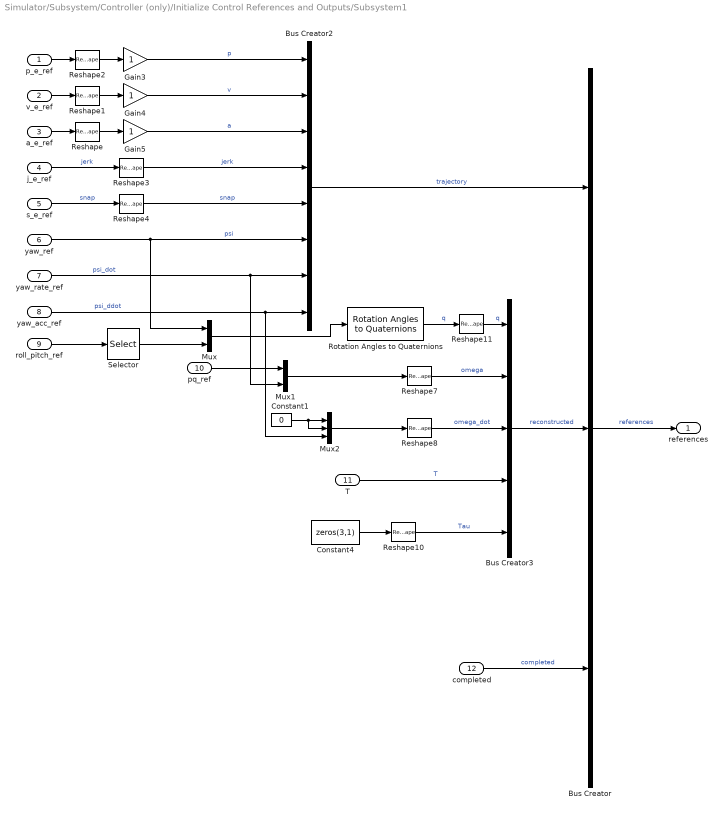
== system Simulator/Subsystem/Controller (only)/Initialize Control References and Outputs/Subsystem1 ==
  p_e_ref : Inport
  v_e_ref : Inport  Port=2
  a_e_ref : Inport  Port=3
  j_e_ref : Inport  Port=4
  s_e_ref : Inport  Port=5
  yaw_ref : Inport  Port=6
  yaw_rate_ref : Inport  Port=7
  yaw_acc_ref : Inport  Port=8
  roll_pitch_ref : Inport  Port=9
  pq_ref : Inport  Port=10
  T : Inport  Port=11
  completed : Inport  Port=12
  Bus Creator : BusCreator  Inputs=3
  Bus Creator2 : BusCreator  Inputs=8
  Bus Creator3 : BusCreator  Inputs=5
  Constant1 : Constant  Value=0
  Constant4 : Constant  Value=zeros(3,1)
  Gain3 : Gain
  Gain4 : Gain
  Gain5 : Gain
  Mux : Mux  Inputs=2
  Mux1 : Mux  Inputs=2
  Mux2 : Mux  Inputs=3
  Reshape{,1..4,7..8,10} (8 alike) : Reshape  OutputDimensionality=Column vector (2-D)
  Reshape11 : Reshape  OutputDimensionality=Row vector (2-D)
  Rotation Angles to Quaternions : sharedtransform/Rotation Angles to Quaternions  rotationOrder=ZYX  aMode=aMode
  Selector : Selector  InputPortWidth=2  IndexOptions=Index vector (dialog)  Indices=[2 1]  OutputSizes=1
  references : Outport
  wires:
  completed/1 -> Bus Creator/3  "completed"
  Constant1/1 -> Mux2/1, Mux2/2
  Mux1/1 -> Reshape7/1
  Selector/1 -> Mux/2
  roll_pitch_ref/1 -> Selector/1
  Mux/1 -> Rotation Angles to Quaternions/1
  Reshape10/1 -> Bus Creator3/5  "Tau"
  Mux2/1 -> Reshape8/1
  Bus Creator2/1 -> Bus Creator/1  "trajectory"
  Bus Creator3/1 -> Bus Creator/2  "reconstructed"
  a_e_ref/1 -> Reshape/1
  v_e_ref/1 -> Reshape1/1
  Reshape11/1 -> Bus Creator3/1  "q"
  Reshape8/1 -> Bus Creator3/3  "omega_dot"
  Rotation Angles to Quaternions/1 -> Reshape11/1  "q"
  Reshape7/1 -> Bus Creator3/2  "omega"
  T/1 -> Bus Creator3/4  "T"
  Bus Creator/1 -> references/1  "references"
  pq_ref/1 -> Mux1/1
  Constant4/1 -> Reshape10/1
  yaw_acc_ref/1 -> Bus Creator2/8, Mux2/3  "psi_ddot"
  yaw_rate_ref/1 -> Bus Creator2/7, Mux1/2  "psi_dot"
  Gain4/1 -> Bus Creator2/2  "v"
  yaw_ref/1 -> Mux/1, Bus Creator2/6  "psi"
  s_e_ref/1 -> Reshape4/1  "snap"
  j_e_ref/1 -> Reshape3/1  "jerk"
  Gain5/1 -> Bus Creator2/3  "a"
  Gain3/1 -> Bus Creator2/1  "p"
  p_e_ref/1 -> Reshape2/1
  Reshape/1 -> Gain5/1
  Reshape1/1 -> Gain4/1
  Reshape2/1 -> Gain3/1
  Reshape3/1 -> Bus Creator2/4  "jerk"
  Reshape4/1 -> Bus Creator2/5  "snap"

== system Simulator/Guidance/Subsystem2/minimum_snap/Subsystem/re-solve trajectory ==
  guidance_active : Inport
  time_since_start_of_traj : Inport  Port=2
  Trajectory : Inport  Port=3
  States : Inport  Port=4
  waypoints_offset_0 : Inport  Port=5
  Enabled Subsystem1 : Subsystem  TreatAsAtomicUnit=on
  trajectory : Outport
  wires:
  Trajectory/1 -> Enabled Subsystem1/3(Trajectory)
  States/1 -> Enabled Subsystem1/4(States)
  Enabled Subsystem1/1(trajectory) -> trajectory/1
  waypoints_offset_0/1 -> Enabled Subsystem1/5(waypoints_offset_0)
  time_since_start_of_traj/1 -> Enabled Subsystem1/2(time_since_start_of_traj)
  guidance_active/1 -> Enabled Subsystem1/1(guidance_active)

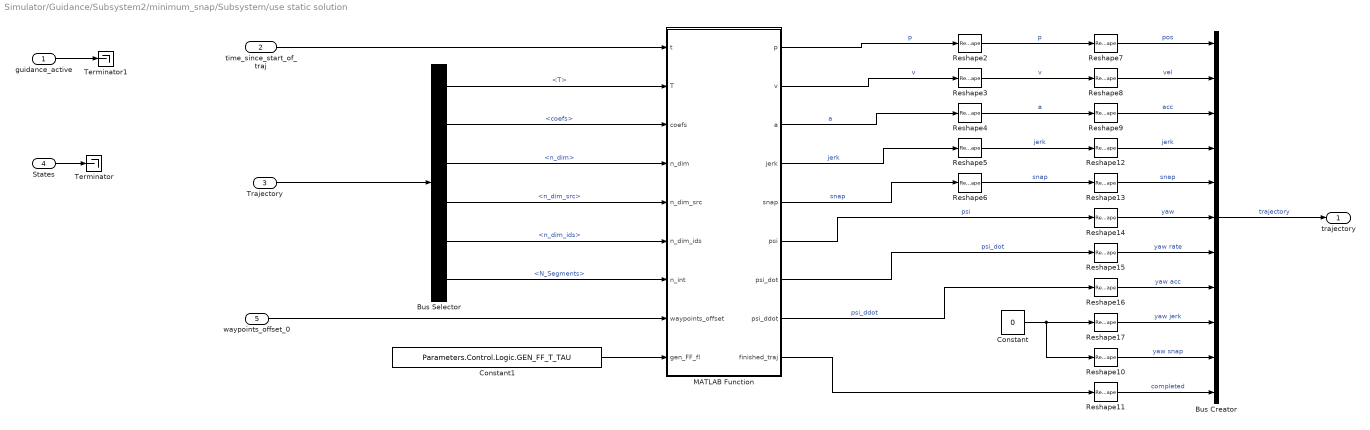
== system Simulator/Guidance/Subsystem2/minimum_snap/Subsystem/use static solution ==
  guidance_active : Inport
  time_since_start_of_traj : Inport  Port=2
  Trajectory : Inport  Port=3
  States : Inport  Port=4
  waypoints_offset_0 : Inport  Port=5
  Bus Creator : BusCreator  Inputs=11
  Bus Selector : BusSelector  OutputSignals=T,coefs,n_dim,n_dim_src,n_dim_ids,N_Segments
  Constant : Constant  Value=0
  Constant1 : Constant  Value=Parameters.Control.Logic.GEN_FF_T_TAU
  MATLAB Function : MATLAB Function  TreatAsAtomicUnit=on
  Reshape{7..17} (11 alike) : Reshape
  Reshape{2..6} (5 alike) : Reshape  OutputDimensionality=Column vector (2-D)
  Terminator : Terminator
  Terminator1 : Terminator
  trajectory : Outport
  wires:
  States/1 -> Terminator/1
  guidance_active/1 -> Terminator1/1
  Bus Selector/1 -> MATLAB Function/2(T)  "<T>"
  Bus Selector/4 -> MATLAB Function/5(n_dim_src)  "<n_dim_src>"
  MATLAB Function/1(p) -> Reshape2/1  "p"
  waypoints_offset_0/1 -> MATLAB Function/8(waypoints_offset)
  MATLAB Function/5(snap) -> Reshape6/1  "snap"
  Trajectory/1 -> Bus Selector/1
  time_since_start_of_traj/1 -> MATLAB Function/1(t)
  Reshape9/1 -> Bus Creator/3  "acc"
  MATLAB Function/4(jerk) -> Reshape5/1  "jerk"
  Bus Selector/6 -> MATLAB Function/7(n_int)  "<N_Segments>"
  MATLAB Function/8(psi_ddot) -> Reshape16/1  "psi_ddot"
  MATLAB Function/3(a) -> Reshape4/1  "a"
  Reshape7/1 -> Bus Creator/1  "pos"
  Reshape4/1 -> Reshape9/1  "a"
  Reshape10/1 -> Bus Creator/10  "yaw snap"
  Bus Selector/3 -> MATLAB Function/4(n_dim)  "<n_dim>"
  Reshape17/1 -> Bus Creator/9  "yaw jerk"
  Reshape15/1 -> Bus Creator/7  "yaw rate"
  Reshape3/1 -> Reshape8/1  "v"
  Reshape13/1 -> Bus Creator/5  "snap"
  Reshape2/1 -> Reshape7/1  "p"
  MATLAB Function/9(finished_traj) -> Reshape11/1
  Reshape8/1 -> Bus Creator/2  "vel"
  Bus Selector/5 -> MATLAB Function/6(n_dim_ids)  "<n_dim_ids>"
  MATLAB Function/2(v) -> Reshape3/1  "v"
  Reshape12/1 -> Bus Creator/4  "jerk"
  MATLAB Function/7(psi_dot) -> Reshape15/1  "psi_dot"
  Bus Creator/1 -> trajectory/1  "trajectory"
  Reshape5/1 -> Reshape12/1  "jerk"
  Reshape6/1 -> Reshape13/1  "snap"
  MATLAB Function/6(psi) -> Reshape14/1  "psi"
  Reshape14/1 -> Bus Creator/6  "yaw"
  Constant/1 -> Reshape10/1, Reshape17/1
  Reshape16/1 -> Bus Creator/8  "yaw acc"
  Reshape11/1 -> Bus Creator/11  "completed"
  Bus Selector/2 -> MATLAB Function/3(coefs)  "<coefs>"
  Constant1/1 -> MATLAB Function/9(gen_FF_fl)

== system Simulator/Inbound Data/Subsystem3/Trajectory Solution/Call solver/Enabled Subsystem ==
  trajectory_id : Inport
  Enable : EnablePort  PropagateVarSize=During execution
  Bus Creator2 : BusCreator  Inputs=6
  Constant : Constant  Value=4
  Display : Display
  MATLAB Function : MATLAB Function  TreatAsAtomicUnit=on
  Trajectory : Outport
  wires:
  trajectory_id/1 -> MATLAB Function/1(trajectory_id)
  Bus Creator2/1 -> Trajectory/1  "Trajectory"
  MATLAB Function/4(n_dim_ids_new) -> Bus Creator2/5  "n_dim_ids"
  MATLAB Function/3(n_dim_new) -> Bus Creator2/3  "n_dim"
  MATLAB Function/2(pp_new) -> Bus Creator2/2  "coefs"
  MATLAB Function/1(T_new) -> Display/1, Bus Creator2/1  "T"
  MATLAB Function/5(N_segments_new) -> Bus Creator2/6  "N_Segments"
  Constant/1 -> Bus Creator2/4  "n_dim_src"

== system Simulator/Inbound Data/Subsystem4/Subsystem/Subsystem1/Disabled ==
  Constant{,1..3} (4 alike) : Constant  Value=0
  Constant19 : Constant  Value=FLIGHT_MODE
  Constant4 : Constant  Value=true
  Display : Display
  roll_stick : Outport
  pitch_stick : Outport  Port=2
  yaw_stick : Outport  Port=3
  Throttle_stick : Outport  Port=4
  FLIGHT_MODE : Outport  Port=5
  ARMED : Outport  Port=6
  wires:
  Constant3/1 -> Throttle_stick/1  "Throttle_stick"
  Constant1/1 -> pitch_stick/1  "pitch_stick"
  Constant/1 -> roll_stick/1  "roll_stick"
  Constant2/1 -> yaw_stick/1  "yaw_stick"
  Constant19/1 -> FLIGHT_MODE/1, Display/1  "FLIGHT_MODE"
  Constant4/1 -> ARMED/1  "ARMED"

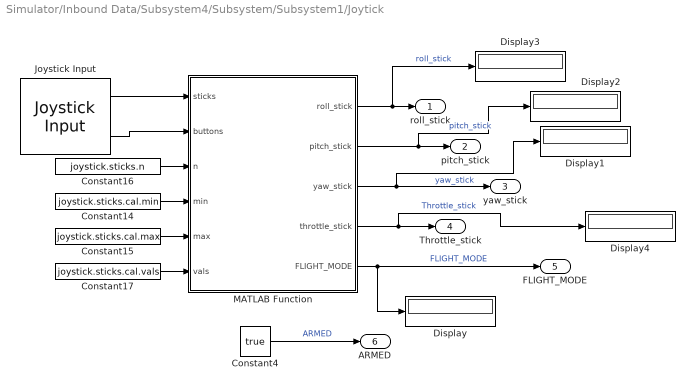
== system Simulator/Inbound Data/Subsystem4/Subsystem/Subsystem1/Joytick ==
  Constant14 : Constant  Value=joystick.sticks.cal.min
  Constant15 : Constant  Value=joystick.sticks.cal.max
  Constant16 : Constant  Value=joystick.sticks.n
  Constant17 : Constant  Value=joystick.sticks.cal.vals
  Constant4 : Constant  Value=true
  Display{,1..4} (5 alike) : Display
  Joystick Input : vrlib/Joystick Input  joyid=1  adjustports=on  forcefeed=off
  MATLAB Function : MATLAB Function  TreatAsAtomicUnit=on
  roll_stick : Outport
  pitch_stick : Outport  Port=2
  yaw_stick : Outport  Port=3
  Throttle_stick : Outport  Port=4
  FLIGHT_MODE : Outport  Port=5
  ARMED : Outport  Port=6
  wires:
  Constant15/1 -> MATLAB Function/5(max)
  Constant14/1 -> MATLAB Function/4(min)
  MATLAB Function/4(throttle_stick) -> Display4/1, Throttle_stick/1  "Throttle_stick"
  Constant16/1 -> MATLAB Function/3(n)
  Constant17/1 -> MATLAB Function/6(vals)
  Joystick Input/1 -> MATLAB Function/1(sticks)
  MATLAB Function/2(pitch_stick) -> Display2/1, pitch_stick/1  "pitch_stick"
  Joystick Input/2 -> MATLAB Function/2(buttons)
  MATLAB Function/1(roll_stick) -> Display3/1, roll_stick/1  "roll_stick"
  MATLAB Function/3(yaw_stick) -> Display1/1, yaw_stick/1  "yaw_stick"
  MATLAB Function/5(FLIGHT_MODE) -> Display/1, FLIGHT_MODE/1  "FLIGHT_MODE"
  Constant4/1 -> ARMED/1  "ARMED"

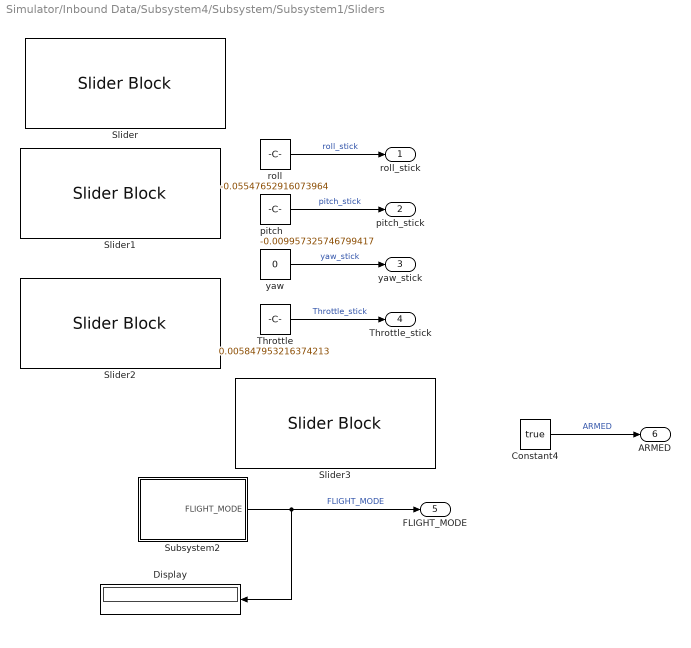
== system Simulator/Inbound Data/Subsystem4/Subsystem/Subsystem1/Sliders ==
  Constant4 : Constant  Value=true
  Display : Display
  Slider{,1..3} (4 alike) : SliderBlock  ScaleMin=-1  ScaleMax=1
  Subsystem2 : Subsystem
  Throttle : Constant  Value=0.005847953216374213
  pitch : Constant  Value=-0.009957325746799417
  roll : Constant  Value=-0.05547652916073964
  yaw : Constant  Value=0
  roll_stick : Outport
  pitch_stick : Outport  Port=2
  yaw_stick : Outport  Port=3
  Throttle_stick : Outport  Port=4
  FLIGHT_MODE : Outport  Port=5
  ARMED : Outport  Port=6
  wires:
  roll/1 -> roll_stick/1  "roll_stick"
  yaw/1 -> yaw_stick/1  "yaw_stick"
  pitch/1 -> pitch_stick/1  "pitch_stick"
  Throttle/1 -> Throttle_stick/1  "Throttle_stick"
  Subsystem2/1(FLIGHT_MODE) -> FLIGHT_MODE/1, Display/1  "FLIGHT_MODE"
  Constant4/1 -> ARMED/1  "ARMED"

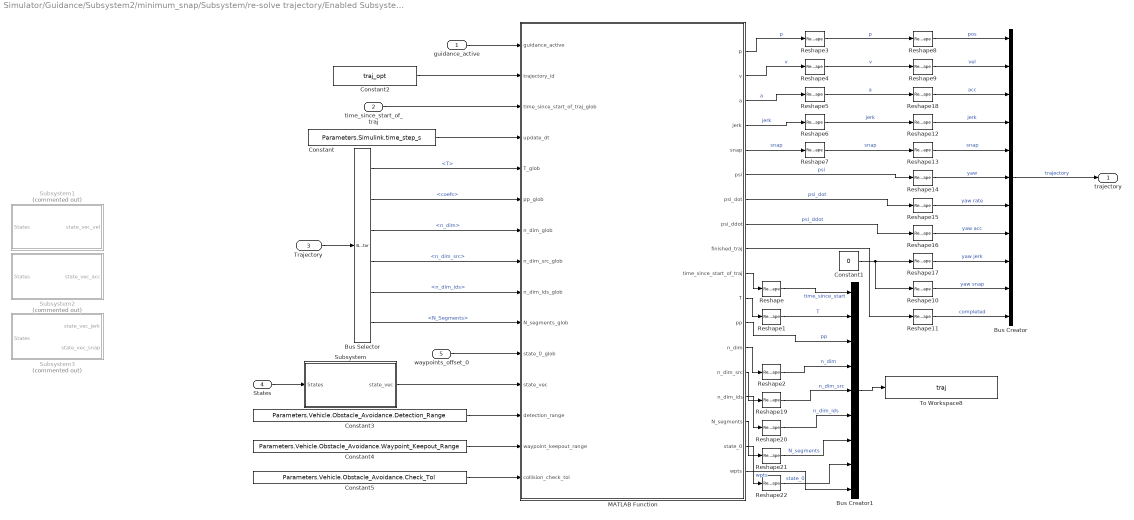
== system Simulator/Guidance/Subsystem2/minimum_snap/Subsystem/re-solve trajectory/Enabled Subsystem1 ==
  guidance_active : Inport
  time_since_start_of_traj : Inport  Port=2
  Trajectory : Inport  Port=3
  States : Inport  Port=4
  waypoints_offset_0 : Inport  Port=5
  Bus Creator : BusCreator  Inputs=11
  Bus Creator1 : BusCreator  Inputs=9
  Bus Selector : BusSelector  OutputSignals=T,coefs,n_dim,n_dim_src,n_dim_ids,N_Segments
  Constant : Constant  Value=Parameters.Simulink.time_step_s
  Constant1 : Constant  Value=0
  Constant2 : Constant  Value=traj_opt
  Constant3 : Constant  Value=Parameters.Vehicle.Obstacle_Avoidance.Detection_Range
  Constant4 : Constant  Value=Parameters.Vehicle.Obstacle_Avoidance.Waypoint_Keepout_Range
  Constant5 : Constant  Value=Parameters.Vehicle.Obstacle_Avoidance.Check_Tol
  MATLAB Function : MATLAB Function  TreatAsAtomicUnit=on
  Reshape{,1..2,8..22} (18 alike) : Reshape
  Reshape{3..7} (5 alike) : Reshape  OutputDimensionality=Column vector (2-D)
  Subsystem : Subsystem
  Subsystem1 : Subsystem  Commented=on
  Subsystem2 : Subsystem  Commented=on
  Subsystem3 : Subsystem  Commented=on
  To Workspace8 : ToWorkspace  VariableName=traj  SaveFormat=Timeseries  SampleTime=-1
      settings: Save2DSignal=2-D array (concatenate along first dimension)
  trajectory : Outport
  wires:
  Trajectory/1 -> Bus Selector/1
  Constant2/1 -> MATLAB Function/2(trajectory_id)
  waypoints_offset_0/1 -> MATLAB Function/11(state_0_glob)
  Bus Selector/1 -> MATLAB Function/5(T_glob)  "<T>"
  Bus Selector/2 -> MATLAB Function/6(pp_glob)  "<coefs>"
  Bus Selector/3 -> MATLAB Function/7(n_dim_glob)  "<n_dim>"
  time_since_start_of_traj/1 -> MATLAB Function/3(time_since_start_of_traj_glob)
  Bus Selector/4 -> MATLAB Function/8(n_dim_src_glob)  "<n_dim_src>"
  Bus Selector/5 -> MATLAB Function/9(n_dim_ids_glob)  "<n_dim_ids>"
  Bus Selector/6 -> MATLAB Function/10(N_segments_glob)  "<N_Segments>"
  guidance_active/1 -> MATLAB Function/1(guidance_active)
  Constant/1 -> MATLAB Function/4(update_dt)
  Reshape3/1 -> Reshape8/1  "p"
  Reshape12/1 -> Bus Creator/4  "jerk"
  MATLAB Function/2(v) -> Reshape4/1  "v"
  Reshape9/1 -> Bus Creator/2  "vel"
  MATLAB Function/1(p) -> Reshape3/1  "p"
  Reshape17/1 -> Bus Creator/9  "yaw jerk"
  Reshape13/1 -> Bus Creator/5  "snap"
  Reshape4/1 -> Reshape9/1  "v"
  Reshape11/1 -> Bus Creator/11  "completed"
  Reshape6/1 -> Reshape12/1  "jerk"
  Reshape14/1 -> Bus Creator/6  "yaw"
  MATLAB Function/6(psi) -> Reshape14/1  "psi"
  Reshape16/1 -> Bus Creator/8  "yaw acc"
  Reshape15/1 -> Bus Creator/7  "yaw rate"
  Reshape7/1 -> Reshape13/1  "snap"
  Constant1/1 -> Reshape10/1, Reshape17/1
  MATLAB Function/9(finished_traj) -> Reshape11/1
  MATLAB Function/8(psi_ddot) -> Reshape16/1  "psi_ddot"
  MATLAB Function/4(jerk) -> Reshape6/1  "jerk"
  MATLAB Function/7(psi_dot) -> Reshape15/1  "psi_dot"
  Reshape5/1 -> Reshape18/1  "a"
  Reshape10/1 -> Bus Creator/10  "yaw snap"
  Bus Creator/1 -> trajectory/1  "trajectory"
  Reshape8/1 -> Bus Creator/1  "pos"
  MATLAB Function/3(a) -> Reshape5/1  "a"
  MATLAB Function/5(snap) -> Reshape7/1  "snap"
  Reshape18/1 -> Bus Creator/3  "acc"
  MATLAB Function/10(time_since_start_of_traj) -> Reshape/1
  MATLAB Function/11(T) -> Reshape1/1
  Reshape/1 -> Bus Creator1/1  "time_since_start"
  Reshape1/1 -> Bus Creator1/2  "T"
  MATLAB Function/13(n_dim) -> Reshape2/1
  MATLAB Function/14(n_dim_src) -> Reshape19/1
  MATLAB Function/15(n_dim_ids) -> Reshape20/1
  MATLAB Function/16(N_segments) -> Reshape21/1
  MATLAB Function/17(state_0) -> Reshape22/1
  Bus Creator1/1 -> To Workspace8/1
  MATLAB Function/12(pp) -> Bus Creator1/3  "pp"
  Reshape2/1 -> Bus Creator1/4  "n_dim"
  Reshape19/1 -> Bus Creator1/5  "n_dim_src"
  Reshape20/1 -> Bus Creator1/6  "n_dim_ids"
  Reshape21/1 -> Bus Creator1/7  "N_segments"
  Reshape22/1 -> Bus Creator1/8  "state_0"
  States/1 -> Subsystem/1(States)
  Subsystem/1(state_vec) -> MATLAB Function/12(state_vec)
  Constant3/1 -> MATLAB Function/13(detection_range)
  Constant4/1 -> MATLAB Function/14(waypoint_keepout_range)
  Constant5/1 -> MATLAB Function/15(collision_check_tol)
  MATLAB Function/18(wpts) -> Bus Creator1/9  "wpts"

== system Simulator/Inbound Data/Subsystem4/Subsystem/Subsystem1/Sliders/Subsystem2 ==
  Constant19 : Constant  Value=FLIGHT_MODE
  Constant3 : Constant  Value=flight_mode.autonomous
  Equal : RelationalOperator  Operator===  OutDataTypeStr=boolean  RndMeth=Simplest  InputSameDT=off
  If : If  IfExpression=u1
  If Action Subsystem : Subsystem  TreatAsAtomicUnit=on
  If Action Subsystem1 : Subsystem  TreatAsAtomicUnit=on
  Merge : Merge
  FLIGHT_MODE : Outport
  wires:
  If/1 -> If Action Subsystem/Action
  If Action Subsystem1/1(Out1) -> Merge/2
  Merge/1 -> FLIGHT_MODE/1
  Constant19/1 -> If Action Subsystem1/1(In1), Equal/1  "FLIGHT_MODE"
  Constant3/1 -> Equal/2
  Equal/1 -> If/1
  If/2 -> If Action Subsystem1/Action
  If Action Subsystem/1(Out1) -> Merge/1

== system Simulator/Guidance/Subsystem2/minimum_snap/Subsystem/re-solve trajectory/Enabled Subsystem1/Subsystem ==
  States : Inport
  Bus Selector2 : BusSelector  OutputSignals=p_e,att
  Mux : Mux  Inputs=2
  Reshape : Reshape
  Reshape1 : Reshape
  Selector : Selector  InputPortWidth=3  IndexOptions=Index vector (dialog)  Indices=[3]  OutputSizes=1
  state_vec : Outport
  wires:
  Mux/1 -> state_vec/1
  States/1 -> Bus Selector2/1
  Reshape/1 -> Mux/1
  Bus Selector2/2 -> Selector/1  "<att>"
  Selector/1 -> Reshape1/1
  Reshape1/1 -> Mux/2
  Bus Selector2/1 -> Reshape/1  "<p_e>"

== system Simulator/Guidance/Subsystem2/minimum_snap/Subsystem/re-solve trajectory/Enabled Subsystem1/Subsystem1 ==
  States : Inport
  Bus Selector2 : BusSelector  OutputSignals=v_e,omega
  Mux : Mux  Inputs=2
  Reshape : Reshape
  Reshape1 : Reshape
  Selector : Selector  InputPortWidth=3  IndexOptions=Index vector (dialog)  Indices=[3]  OutputSizes=1
  state_vec_vel : Outport
  wires:
  Mux/1 -> state_vec_vel/1
  States/1 -> Bus Selector2/1
  Reshape/1 -> Mux/1
  Bus Selector2/2 -> Selector/1  "<omega>"
  Selector/1 -> Reshape1/1
  Reshape1/1 -> Mux/2
  Bus Selector2/1 -> Reshape/1  "<v_e>"

== system Simulator/Guidance/Subsystem2/minimum_snap/Subsystem/re-solve trajectory/Enabled Subsystem1/Subsystem2 ==
  States : Inport
  Bus Selector2 : BusSelector  OutputSignals=a_e,omega_dot
  Mux : Mux  Inputs=2
  Reshape : Reshape
  Reshape1 : Reshape
  Selector : Selector  InputPortWidth=3  IndexOptions=Index vector (dialog)  Indices=[3]  OutputSizes=1
  state_vec_acc : Outport
  wires:
  Mux/1 -> state_vec_acc/1
  States/1 -> Bus Selector2/1
  Reshape/1 -> Mux/1
  Bus Selector2/2 -> Selector/1  "<omega_dot>"
  Selector/1 -> Reshape1/1
  Reshape1/1 -> Mux/2
  Bus Selector2/1 -> Reshape/1  "<a_e>"
